simulink model "Observer"  (R2018b)
settings: Solver=VariableStepAuto  StartTime=0.0  StopTime=10.0  RelTol=1e-3
undefined symbols (not defined in the file): A_obs, B_obs, DiscIntNeverNeededParam, K_new, L
libraries: legoev3lib x2
settings Model: Creator=stinu  LastModifiedBy=stinu

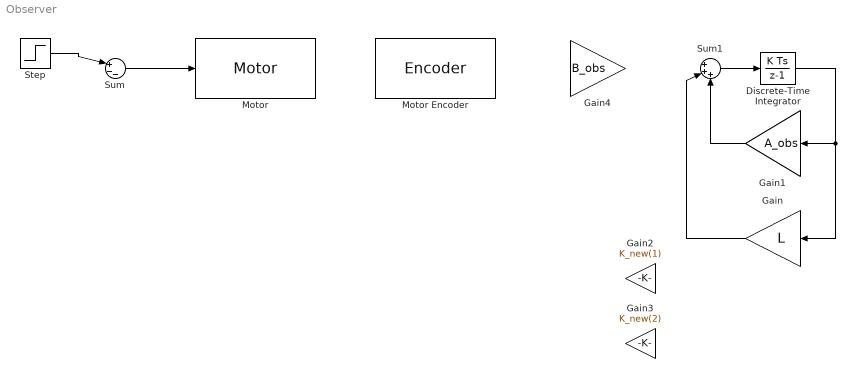
== system Observer ==
  Discrete-Time Integrator : DiscreteIntegrator  SampleTime=-1  ICPrevOutput=DiscIntNeverNeededParam  ICPrevScaledInput=DiscIntNeverNeededParam
  Gain : Gain  Gain=L
  Gain1 : Gain  Gain=A_obs
  Gain2 : Gain  Gain=K_new(1)
  Gain3 : Gain  Gain=K_new(2)
  Gain4 : Gain  Gain=B_obs
  Motor : legoev3lib/Motor  sportNumber=A  sstopAction=Brake
  Motor Encoder : legoev3lib/Encoder  portNumber=A  opMode=No reset  sampleTime=0.01
      settings: SourceProductName=Simulink Support Package for LEGO MINDSTORMS EV3 Hardware  SourceProductBaseCode=LEGOEV3
  Step : Step  After=-100  SampleTime=0.01
  Sum : Sum  Inputs=|+--
  Sum1 : Sum  Inputs=|+++
  wires:
  Step/1 -> Sum/1
  Sum/1 -> Motor/1
  Gain1/1 -> Sum1/3
  Sum1/1 -> Discrete-Time Integrator/1
  Discrete-Time Integrator/1 -> Gain/1, Gain1/1
  Gain/1 -> Sum1/2
